simulink model "InverseDynamics"  (R2014a)
settings: Solver=ode45  StartTime=0.0  StopTime=inf  RelTol=1e-3
libraries: m3dof_library x10
settings Model: Creator=diego  LastModifiedBy=diego

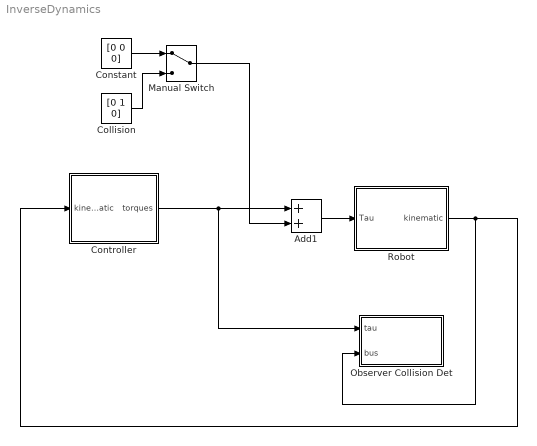
== system InverseDynamics ==
  Add1 : Sum
  Collision : Constant  Value=[0 1 0]
  Constant : Constant  Value=[0 0 0]
  Controller : Subsystem
  Manual Switch : ManualSwitch
  Observer Collision Det : Subsystem
  Robot : Subsystem
  wires:
  Controller/1(torques) -> Observer Collision Det/1(tau), Add1/1
  Robot/1(kinematic) -> Observer Collision Det/2(bus), Controller/1(kinematic)
  Add1/1 -> Robot/1(Tau)
  Constant/1 -> Manual Switch/1
  Collision/1 -> Manual Switch/2
  Manual Switch/1 -> Add1/2

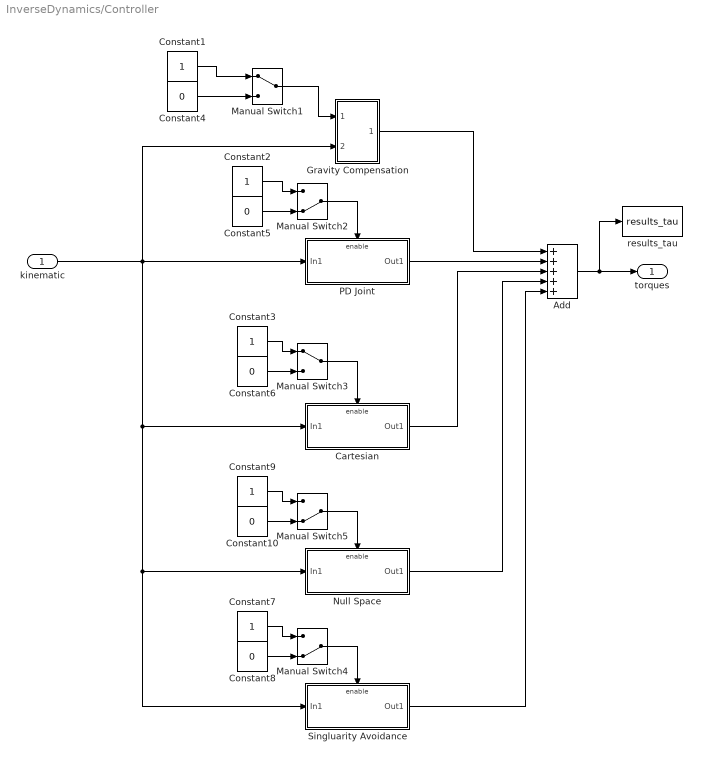
== system InverseDynamics/Controller ==
  kinematic : Inport
  Add : Sum  Inputs=+++++
  Cartesian : Subsystem  TreatAsAtomicUnit=on
  Constant{1..3,7,9} (5 alike) : Constant
  Constant{5..6,8,10} (4 alike) : Constant  Value=0
  Constant4 : Constant  Value=0  VectorParams1D=off
  Gravity Compensation : Subsystem
  Manual Switch1 : ManualSwitch
  Manual Switch2 : ManualSwitch  CurrentSetting=0
  Manual Switch3 : ManualSwitch
  Manual Switch4 : ManualSwitch  CurrentSetting=0
  Manual Switch5 : ManualSwitch  CurrentSetting=0
  Null Space : Subsystem  TreatAsAtomicUnit=on
  PD Joint : Subsystem  TreatAsAtomicUnit=on
  Singluarity Avoidance : Subsystem  TreatAsAtomicUnit=on
  results_tau : ToWorkspace  VariableName=results_tau  SaveFormat=Timeseries  SampleTime=-1
  torques : Outport
  wires:
  Constant1/1 -> Manual Switch1/1
  Constant2/1 -> Manual Switch2/1
  PD Joint/1(Out1) -> Add/2
  Manual Switch3/1 -> Cartesian/Enable
  Cartesian/1(Out1) -> Add/3
  Constant3/1 -> Manual Switch3/1
  Constant6/1 -> Manual Switch3/2
  Manual Switch2/1 -> PD Joint/Enable
  Add/1 -> results_tau/1, torques/1
  Constant5/1 -> Manual Switch2/2
  kinematic/1 -> Gravity Compensation/2(bus), Cartesian/1(In1), Null Space/1(In1), Singluarity Avoidance/1(In1), PD Joint/1(In1)
  Manual Switch4/1 -> Singluarity Avoidance/Enable
  Constant7/1 -> Manual Switch4/1
  Constant8/1 -> Manual Switch4/2
  Manual Switch5/1 -> Null Space/Enable
  Constant9/1 -> Manual Switch5/1
  Constant10/1 -> Manual Switch5/2
  Null Space/1(Out1) -> Add/4
  Singluarity Avoidance/1(Out1) -> Add/5
  Constant4/1 -> Manual Switch1/2
  Manual Switch1/1 -> Gravity Compensation/1(activation)
  Gravity Compensation/1(tau_g) -> Add/1

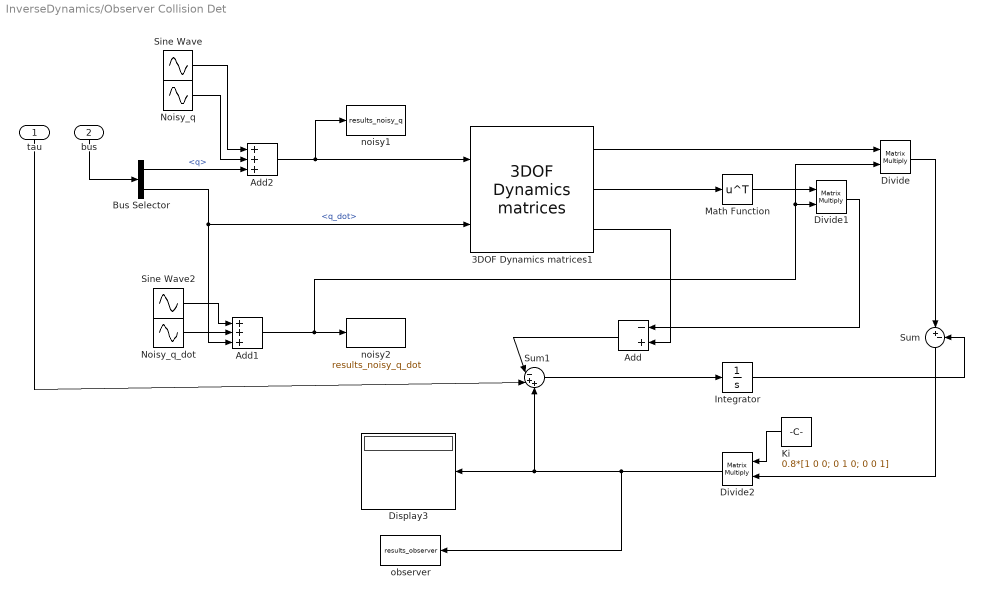
== system InverseDynamics/Observer Collision Det ==
  tau : Inport
  bus : Inport  Port=2
  3DOF Dynamics matrices1 : m3dof_library/3DOF Dynamics matrices  m1=m1  mX1=mx1  ZZ1=I1  m2=m2  mX2=mx2  ZZ2=I2  m3=m3  mX3=mx3  ZZ3=I3  a1=l1  a2=l2  a3=l3  eg=eg
  Add : Sum  Inputs=-+
  Add1 : Sum  Inputs=+++
  Add2 : Sum  Inputs=+++
  Bus Selector : BusSelector  OutputSignals=q,q_dot
  Display3 : Display
  Divide : Product  Inputs=**  Multiplication=Matrix(*)
  Divide1 : Product  Inputs=**  Multiplication=Matrix(*)
  Divide2 : Product  Inputs=**  Multiplication=Matrix(*)
  Integrator : Integrator
  Ki : Constant  Value=0.8*[1 0 0; 0 1 0; 0 0 1]
  Math Function : Math  Operator=transpose  SaturateOnIntegerOverflow=on
  Noisy_q : Sin  Amplitude=0.01  Frequency=10000000  SampleTime=0
  Noisy_q_dot : Sin  Amplitude=0.02  Frequency=500000  SampleTime=0
  Sine Wave : Sin  Amplitude=0.002  Frequency=1000000  SampleTime=0
  Sine Wave2 : Sin  Amplitude=0.01  Frequency=2000000  SampleTime=0
  Sum : Sum  Inputs=|+-
  Sum1 : Sum  Inputs=|-++
  noisy1 : ToWorkspace  VariableName=results_noisy_q  SaveFormat=Timeseries  SampleTime=-1
  noisy2 : ToWorkspace  VariableName=results_noisy_q_dot  SaveFormat=Timeseries  SampleTime=-1
  observer : ToWorkspace  VariableName=results_observer  SaveFormat=Timeseries  SampleTime=-1
  wires:
  bus/1 -> Bus Selector/1
  tau/1 -> Sum1/2
  3DOF Dynamics matrices1/1 -> Divide/1
  Divide/1 -> Sum/1
  3DOF Dynamics matrices1/2 -> Math Function/1
  Math Function/1 -> Divide1/1
  Divide1/1 -> Add/1
  3DOF Dynamics matrices1/3 -> Add/2
  Add/1 -> Sum1/1
  Sum1/1 -> Integrator/1
  Integrator/1 -> Sum/2
  Ki/1 -> Divide2/1
  Sum/1 -> Divide2/2
  Divide2/1 -> observer/1, Sum1/3, Display3/1
  Sine Wave/1 -> Add2/1
  Noisy_q/1 -> Add2/2
  Bus Selector/1 -> Add2/3  "<q>"
  Add2/1 -> noisy1/1, 3DOF Dynamics matrices1/1
  Sine Wave2/1 -> Add1/1
  Noisy_q_dot/1 -> Add1/2
  Bus Selector/2 -> 3DOF Dynamics matrices1/2, Add1/3  "<q_dot>"
  Add1/1 -> Divide/2, Divide1/2, noisy2/1

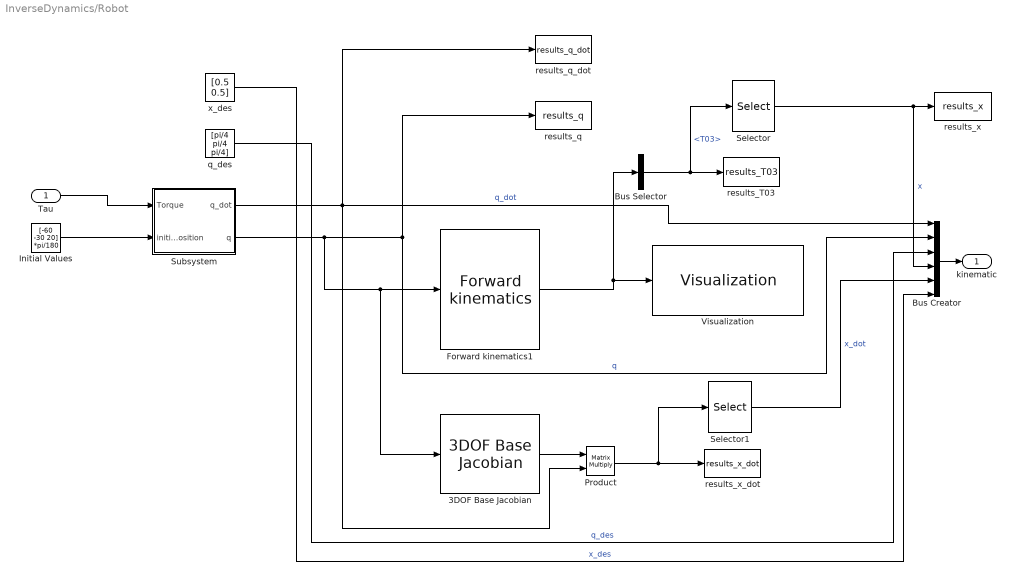
== system InverseDynamics/Robot ==
  Tau : Inport
  3DOF Base Jacobian : m3dof_library/3DOF Base Jacobian  a1=l1  a2=l2  a3=l3
  Bus Creator : BusCreator  Inputs='q_dot','q','q_des','x','x_dot','x_des'
  Bus Selector : BusSelector  OutputSignals=T03
  Forward kinematics1 : m3dof_library/Forward kinematics  a1=l1  a2=l2  a3=l3  alpha=0
  Initial Values : Constant  Value=[-60 -30 20] *pi/180
  Product : Product  Multiplication=Matrix(*)
  Selector : Selector  NumberOfDimensions=2  InputPortWidth=2  IndexOptions=Index vector (dialog),Index vector (dialog)  Indices=[1 2],4  OutputSizes=1,1
  Selector1 : Selector  InputPortWidth=3  Indices=[1 2]
  Subsystem : Subsystem
  Visualization : m3dof_library/Visualization  Ts0=0.01  al=1  a1=l1  a2=l2  a3=l3  alpha=0  eg=eg  tl=50
  q_des : Constant  Value=[pi/4 pi/4 pi/4]
  results_T03 : ToWorkspace  VariableName=results_T03  SaveFormat=Timeseries  SampleTime=-1
  results_q : ToWorkspace  VariableName=results_q  SaveFormat=Timeseries  SampleTime=-1
  results_q_dot : ToWorkspace  VariableName=results_q_dot  SaveFormat=Timeseries  SampleTime=-1
  results_x : ToWorkspace  VariableName=results_x  SaveFormat=Timeseries  SampleTime=-1
  results_x_dot : ToWorkspace  VariableName=results_x_dot  SaveFormat=Timeseries  SampleTime=-1
  x_des : Constant  Value=[0.5 0.5]
  kinematic : Outport
  wires:
  Tau/1 -> Subsystem/1(Torque)
  Initial Values/1 -> Subsystem/2(initial_position)
  Forward kinematics1/1 -> Bus Selector/1, Visualization/1
  3DOF Base Jacobian/1 -> Product/1
  Product/1 -> Selector1/1, results_x_dot/1
  Bus Selector/1 -> Selector/1, results_T03/1  "<T03>"
  Subsystem/1(q_dot) -> Product/2, results_q_dot/1, Bus Creator/1  "q_dot"
  Subsystem/2(q) -> 3DOF Base Jacobian/1, Forward kinematics1/1, results_q/1, Bus Creator/2  "q"
  q_des/1 -> Bus Creator/3  "q_des"
  x_des/1 -> Bus Creator/6  "x_des"
  Selector1/1 -> Bus Creator/5  "x_dot"
  Selector/1 -> results_x/1, Bus Creator/4  "x"
  Bus Creator/1 -> kinematic/1

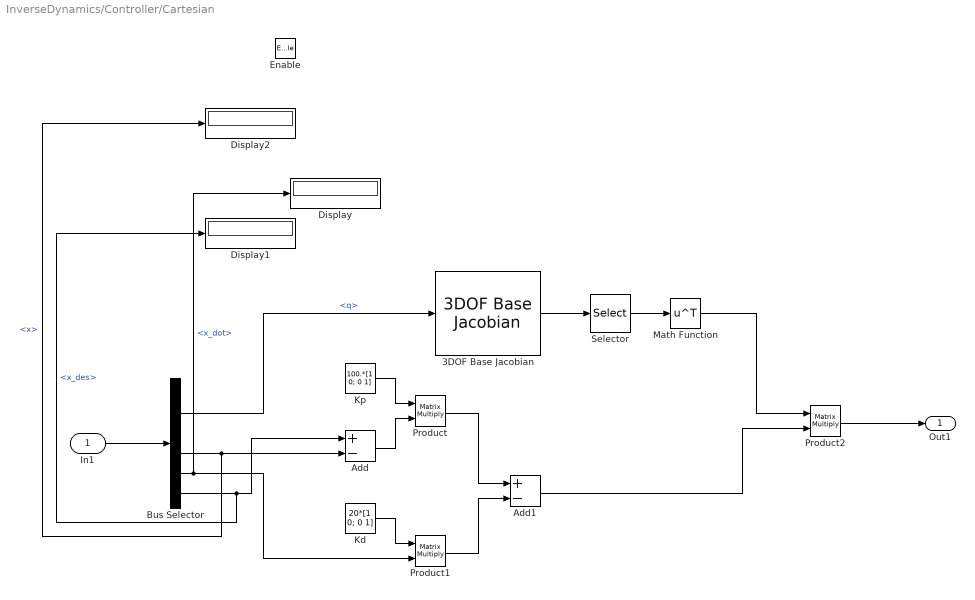
== system InverseDynamics/Controller/Cartesian ==
  In1 : Inport
  Enable : EnablePort
  3DOF Base Jacobian : m3dof_library/3DOF Base Jacobian  a1=l1  a2=l2  a3=l3
  Add : Sum  Inputs=+-
  Add1 : Sum  Inputs=+-
  Bus Selector : BusSelector  OutputSignals=q_dot,q,q_des,x,x_dot,x_des
  Display : Display
  Display1 : Display
  Display2 : Display
  "Kd " : Constant  Value=20*[1 0; 0 1]
  Kp : Constant  Value=100.*[1 0; 0 1]
  Math Function : Math  Operator=transpose  SaturateOnIntegerOverflow=on
  Product : Product  Multiplication=Matrix(*)
  Product1 : Product  Multiplication=Matrix(*)
  Product2 : Product  Multiplication=Matrix(*)
  Selector : Selector  NumberOfDimensions=2  InputPortWidth=3  IndexOptions=Index vector (dialog),Index vector (dialog)  Indices=[1 2],[1 2 3]  OutputSizes=1,1
  Out1 : Outport
  wires:
  In1/1 -> Bus Selector/1
  Kp/1 -> Product/1
  Add/1 -> Product/2
  Product/1 -> Add1/1
  Product1/1 -> Add1/2
  Bus Selector/6 -> Display1/1, Add/1  "<x_des>"
  Bus Selector/4 -> Display2/1, Add/2  "<x>"
  Bus Selector/5 -> Product1/2, Display/1  "<x_dot>"
  "Kd "/1 -> Product1/1
  Bus Selector/2 -> 3DOF Base Jacobian/1  "<q>"
  Product2/1 -> Out1/1
  3DOF Base Jacobian/1 -> Selector/1
  Selector/1 -> Math Function/1
  Math Function/1 -> Product2/1
  Add1/1 -> Product2/2

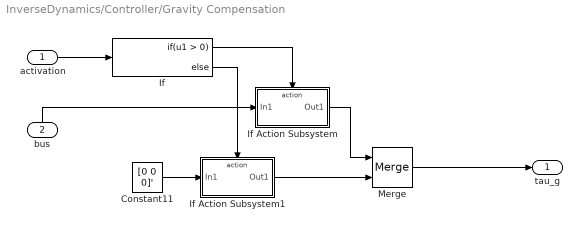
== system InverseDynamics/Controller/Gravity Compensation ==
  activation : Inport
  bus : Inport  Port=2
  Constant11 : Constant  Value=[0 0 0]'  VectorParams1D=off
  If : If
  If Action Subsystem : Subsystem  TreatAsAtomicUnit=on
  If Action Subsystem1 : Subsystem  TreatAsAtomicUnit=on
  Merge : Merge
  tau_g : Outport
  wires:
  bus/1 -> If Action Subsystem/1(In1)
  Constant11/1 -> If Action Subsystem1/1(In1)
  If/2 -> If Action Subsystem1/Action
  If/1 -> If Action Subsystem/Action
  activation/1 -> If/1
  If Action Subsystem1/1(Out1) -> Merge/2
  Merge/1 -> tau_g/1
  If Action Subsystem/1(Out1) -> Merge/1

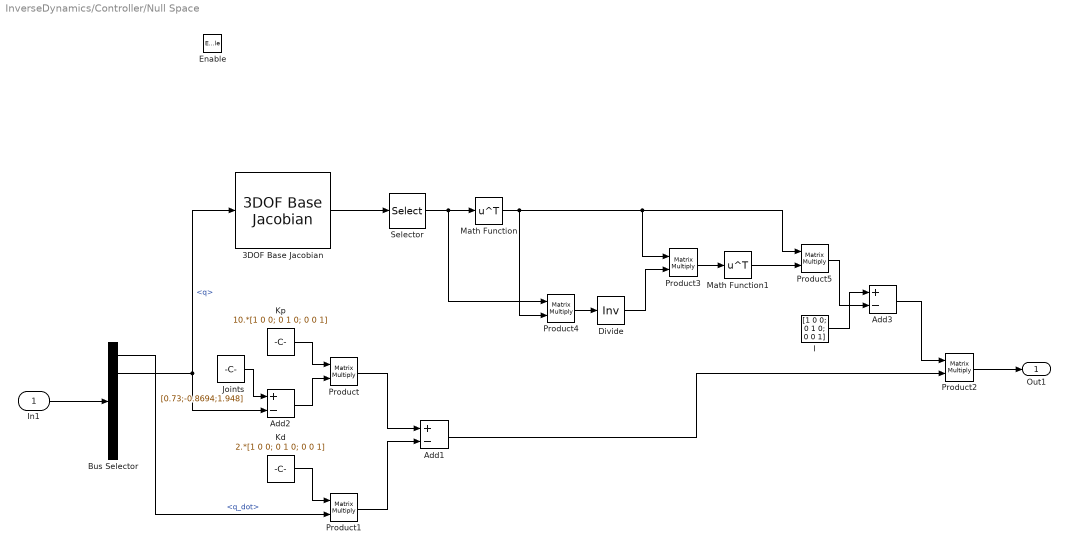
== system InverseDynamics/Controller/Null Space ==
  In1 : Inport
  Enable : EnablePort
  3DOF Base Jacobian : m3dof_library/3DOF Base Jacobian  a1=l1  a2=l2  a3=l3
  Add1 : Sum  Inputs=+-
  Add2 : Sum  Inputs=+-
  Add3 : Sum  Inputs=+-
  Bus Selector : BusSelector  OutputSignals=q_dot,q,q_des,x,x_dot,x_des
  Divide : Product  Inputs=/  Multiplication=Matrix(*)
  I : Constant  Value=[1 0 0; 0 1 0; 0 0 1]
  Joints : Constant  Value=[0.73;-0.8694;1.948]
  "Kd " : Constant  Value=2.*[1 0 0; 0 1 0; 0 0 1]
  Kp : Constant  Value=10.*[1 0 0; 0 1 0; 0 0 1]
  Math Function : Math  Operator=transpose  SaturateOnIntegerOverflow=on
  Math Function1 : Math  Operator=transpose  SaturateOnIntegerOverflow=on
  Product{,1..5} (6 alike) : Product  Multiplication=Matrix(*)
  Selector : Selector  NumberOfDimensions=2  InputPortWidth=3  IndexOptions=Index vector (dialog),Index vector (dialog)  Indices=[1 2],[1 2 3]  OutputSizes=1,1
  Out1 : Outport
  wires:
  Add1/1 -> Product2/2
  Bus Selector/1 -> Product1/2  "<q_dot>"
  Add3/1 -> Product2/1
  Product5/1 -> Add3/2
  I/1 -> Add3/1
  Math Function1/1 -> Product5/2
  Product3/1 -> Math Function1/1
  Divide/1 -> Product3/2
  Product4/1 -> Divide/1
  Joints/1 -> Add2/1
  Add2/1 -> Product/2
  Math Function/1 -> Product5/1, Product3/1, Product4/2
  Selector/1 -> Math Function/1, Product4/1
  3DOF Base Jacobian/1 -> Selector/1
  Product2/1 -> Out1/1
  Bus Selector/2 -> 3DOF Base Jacobian/1, Add2/2  "<q>"
  "Kd "/1 -> Product1/1
  Product1/1 -> Add1/2
  Product/1 -> Add1/1
  Kp/1 -> Product/1
  In1/1 -> Bus Selector/1

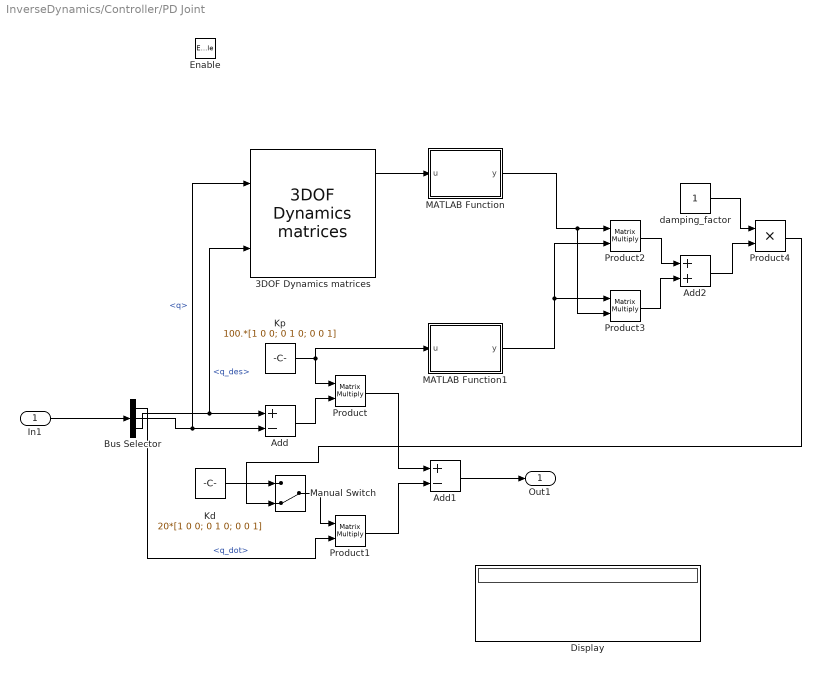
== system InverseDynamics/Controller/PD Joint ==
  In1 : Inport
  Enable : EnablePort  StatesWhenEnabling=reset
  3DOF Dynamics matrices : m3dof_library/3DOF Dynamics matrices  m1=m1  mX1=mx1  ZZ1=I1  m2=m2  mX2=mx2  ZZ2=I2  m3=m3  mX3=mx3  ZZ3=I3  a1=l1  a2=l2  a3=l3  eg=eg
  Add : Sum  Inputs=+-
  Add1 : Sum  Inputs=+-
  Add2 : Sum
  Bus Selector : BusSelector  OutputSignals=q_dot,q,q_des
  Display : Display
  "Kd " : Constant  Value=20*[1 0 0; 0 1 0; 0 0 1]
  Kp : Constant  Value=100.*[1 0 0; 0 1 0; 0 0 1]
  MATLAB Function : MATLAB Function  TreatAsAtomicUnit=on
  MATLAB Function1 : MATLAB Function  TreatAsAtomicUnit=on
  Manual Switch : ManualSwitch  CurrentSetting=0
  Product{,1..3} (4 alike) : Product  Multiplication=Matrix(*)
  Product4 : Product
  damping_factor : Constant
  Out1 : Outport
  wires:
  In1/1 -> Bus Selector/1
  Bus Selector/1 -> Product1/2  "<q_dot>"
  Bus Selector/2 -> 3DOF Dynamics matrices/1, Add/2  "<q>"
  Bus Selector/3 -> 3DOF Dynamics matrices/2, Add/1  "<q_des>"
  Kp/1 -> MATLAB Function1/1(u), Product/1
  Add/1 -> Product/2
  Product/1 -> Add1/1
  Product1/1 -> Add1/2
  Add1/1 -> Out1/1
  Product2/1 -> Add2/1
  Product3/1 -> Add2/2
  3DOF Dynamics matrices/1 -> MATLAB Function/1(u)
  MATLAB Function/1(y) -> Product3/2, Product2/1
  MATLAB Function1/1(y) -> Product2/2, Product3/1
  damping_factor/1 -> Product4/1
  Add2/1 -> Product4/2
  Product4/1 -> Manual Switch/2
  "Kd "/1 -> Manual Switch/1
  Manual Switch/1 -> Product1/1

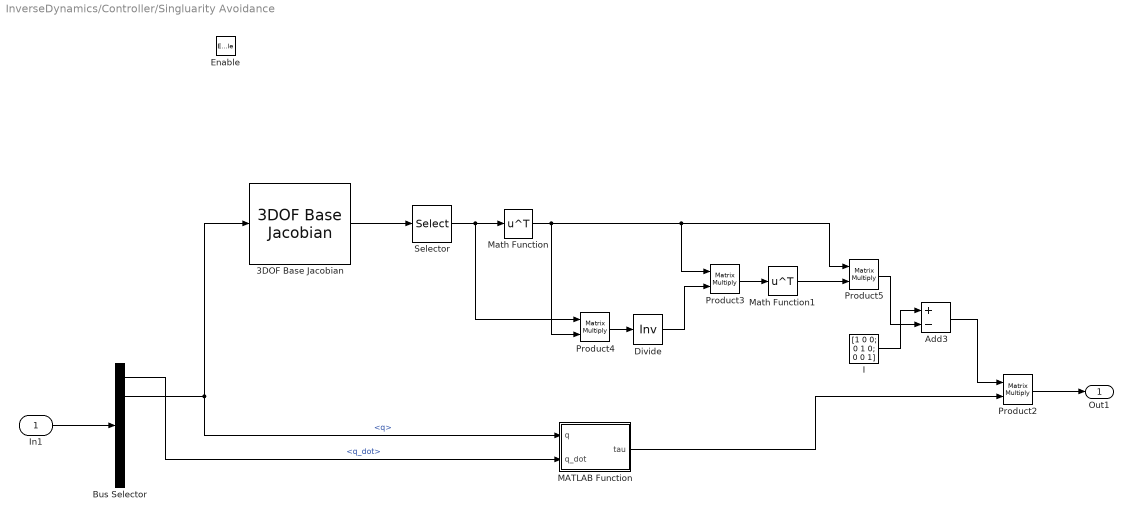
== system InverseDynamics/Controller/Singluarity Avoidance ==
  In1 : Inport
  Enable : EnablePort
  3DOF Base Jacobian : m3dof_library/3DOF Base Jacobian  a1=l1  a2=l2  a3=l3
  Add3 : Sum  Inputs=+-
  Bus Selector : BusSelector  OutputSignals=q_dot,q,q_des,x,x_dot,x_des
  Divide : Product  Inputs=/  Multiplication=Matrix(*)
  I : Constant  Value=[1 0 0; 0 1 0; 0 0 1]
  MATLAB Function : MATLAB Function  TreatAsAtomicUnit=on
  Math Function : Math  Operator=transpose  SaturateOnIntegerOverflow=on
  Math Function1 : Math  Operator=transpose  SaturateOnIntegerOverflow=on
  Product{2..5} (4 alike) : Product  Multiplication=Matrix(*)
  Selector : Selector  NumberOfDimensions=2  InputPortWidth=3  IndexOptions=Index vector (dialog),Index vector (dialog)  Indices=[1 2],[1 2 3]  OutputSizes=1,1
  Out1 : Outport
  wires:
  In1/1 -> Bus Selector/1
  Bus Selector/2 -> 3DOF Base Jacobian/1, MATLAB Function/1(q)  "<q>"
  Product2/1 -> Out1/1
  3DOF Base Jacobian/1 -> Selector/1
  Selector/1 -> Product4/1, Math Function/1
  Math Function/1 -> Product4/2, Product3/1, Product5/1
  Product4/1 -> Divide/1
  Divide/1 -> Product3/2
  Product3/1 -> Math Function1/1
  Math Function1/1 -> Product5/2
  I/1 -> Add3/1
  Product5/1 -> Add3/2
  Add3/1 -> Product2/1
  Bus Selector/1 -> MATLAB Function/2(q_dot)  "<q_dot>"
  MATLAB Function/1(tau) -> Product2/2

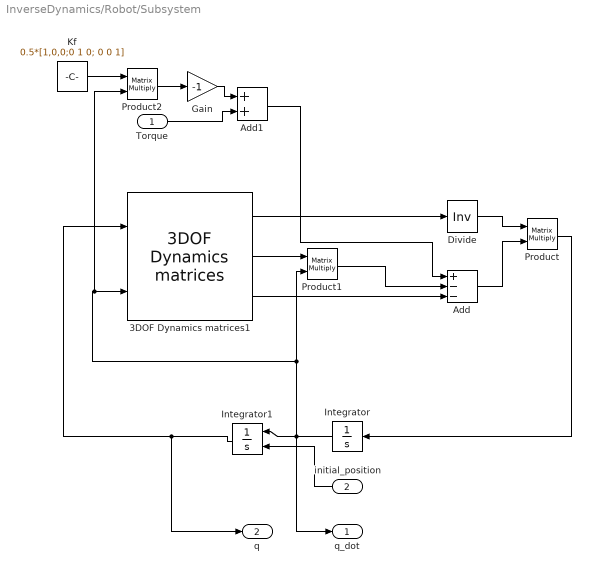
== system InverseDynamics/Robot/Subsystem ==
  Torque : Inport
  initial_position : Inport  Port=2
  3DOF Dynamics matrices1 : m3dof_library/3DOF Dynamics matrices  m1=m1  mX1=mx1  ZZ1=I1  m2=m2  mX2=mx2  ZZ2=I2  m3=m3  mX3=mx3  ZZ3=I3  a1=l1  a2=l2  a3=l3  eg=eg
  Add : Sum  Inputs=+--
  Add1 : Sum
  Divide : Product  Inputs=/  Multiplication=Matrix(*)
  Gain : Gain  Gain=-1
  Integrator : Integrator
  Integrator1 : Integrator  InitialConditionSource=external
  Kf : Constant  Value=0.5*[1,0,0;0 1 0; 0 0 1]
  Product : Product  Multiplication=Matrix(*)
  Product1 : Product  Multiplication=Matrix(*)
  Product2 : Product  Multiplication=Matrix(*)
  q_dot : Outport
  q : Outport  Port=2
  wires:
  Torque/1 -> Add1/2
  Product/1 -> Integrator/1
  Divide/1 -> Product/1
  Add1/1 -> Add/1
  Integrator1/1 -> 3DOF Dynamics matrices1/1, q/1
  Integrator/1 -> q_dot/1, Product2/2, 3DOF Dynamics matrices1/2, Product1/2, Integrator1/1
  Add/1 -> Product/2
  3DOF Dynamics matrices1/1 -> Divide/1
  3DOF Dynamics matrices1/3 -> Add/3
  3DOF Dynamics matrices1/2 -> Product1/1
  Product1/1 -> Add/2
  Kf/1 -> Product2/1
  Product2/1 -> Gain/1
  Gain/1 -> Add1/1
  initial_position/1 -> Integrator1/2

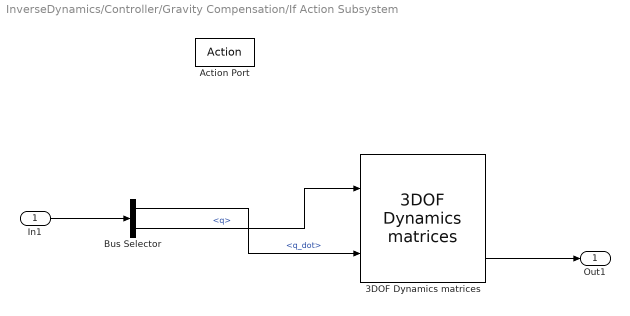
== system InverseDynamics/Controller/Gravity Compensation/If Action Subsystem ==
  In1 : Inport
  Action Port : ActionPort  ActionType=then
  3DOF Dynamics matrices : m3dof_library/3DOF Dynamics matrices  m1=m1  mX1=mx1  ZZ1=I1  m2=m2  mX2=mx2  ZZ2=I2  m3=m3  mX3=mx3  ZZ3=I3  a1=l1  a2=l2  a3=l3  eg=eg
  Bus Selector : BusSelector  OutputSignals=q_dot,q
  Out1 : Outport
  wires:
  3DOF Dynamics matrices/3 -> Out1/1
  In1/1 -> Bus Selector/1
  Bus Selector/1 -> 3DOF Dynamics matrices/2  "<q_dot>"
  Bus Selector/2 -> 3DOF Dynamics matrices/1  "<q>"

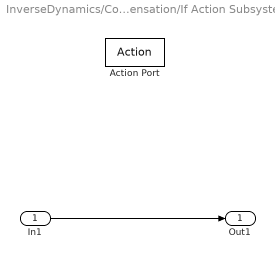
== system InverseDynamics/Controller/Gravity Compensation/If Action Subsystem1 ==
  In1 : Inport
  Action Port : ActionPort  ActionType=else
  Out1 : Outport
  wires:
  In1/1 -> Out1/1

== matlab function InverseDynamics/Controller/PD Joint/MATLAB Function1 ==
  data: u input; y output
function y = fcn(u)
%#codegen

y = real(sqrtm(real(u)));

== matlab function InverseDynamics/Controller/PD Joint/MATLAB Function ==
  data: u input; y output
function y = fcn(u)
%#codegen

y = real(sqrtm(real(u)));

== matlab function InverseDynamics/Controller/Singluarity Avoidance/MATLAB Function ==
  data: q input; tau output; q_dot input
function tau = fcn(q,q_dot)

l1 = 0.1111;
l2 = 0.1111;
% l3 = 0.1111;

m = l1*l2*sin(q);
Jpq = [0 0 0;0 l1*l2*cos(q(2)) 0; 0 0 0];
Kp = 4000*[1 0 0; 0 1 0; 0 0 1];
Kd = 50*[1 0 0; 0 1 0; 0 0 1];

if m(2) < 0.05
    tau = +Jpq'*Kp*(m) + Jpq'*Kd*l1*l2*cos(q(2))*q_dot;
else
    tau = zeros(3,1);
end
